simulink model "DSB_SSB"  (R2023a)
settings: Solver=VariableStepAuto  StartTime=0.0  StopTime=1  RelTol=1e-3
libraries: dspfdesign x2
settings Model: Creator=dung  LastModifiedBy=dung

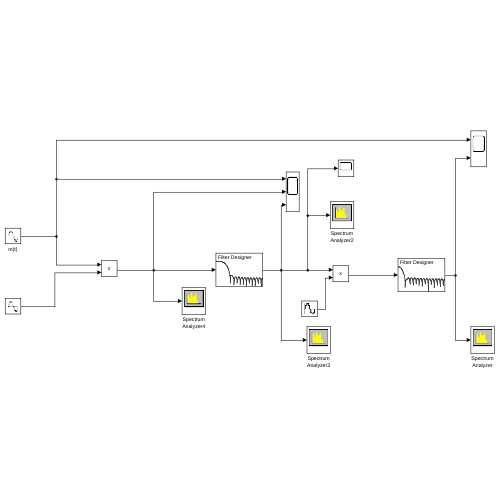
[thumbnail: Simulink's stored preview of the top-level diagram]
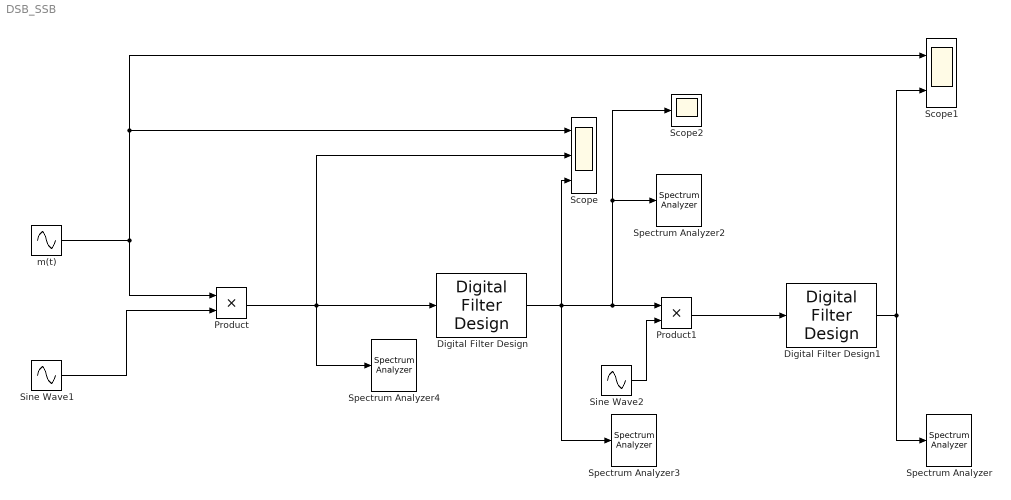
== system DSB_SSB ==
  Digital Filter Design : dspfdesign/Digital Filter Design  mwdsp_browser_bugfix_var=off
  Digital Filter Design1 : dspfdesign/Digital Filter Design  mwdsp_browser_bugfix_var=off
  Product : Product
  Product1 : Product
  Scope : Scope  NumInputPorts=3
  Scope1 : Scope  NumInputPorts=2
  Scope2 : Scope
  Sine Wave1 : Sin  Amplitude=5  Frequency=2*pi*10000  SampleTime=1/100000
  Sine Wave2 : Sin  Frequency=2*pi*10000  SampleTime=1/100000
  Spectrum Analyzer : SpectrumAnalyzer  WindowPosition=[560.000000,290.000000,800.000000,500.000000,]  ScopeFrameLocation=window  YLimits=[-253.6996542,53.22863961]  ColorLimits=[-20 80]  DefaultConfigurationName=spbscopes.SpectrumAnalyzerBlockCfg  IsFrequencyInputMode=0  FrequencyVectorPort=0  FrequencyVectorFromPort=0  FrequencyInputRBWPort=0  FrequencyInputRBWFromPort=0
  Spectrum Analyzer2 : SpectrumAnalyzer  WindowPosition=[562.000000,289.000000,800.000000,500.000000,]  ScopeFrameLocation=window  YLimits=[-248.57224363,56.6885393]  ColorLimits=[-20 80]  DefaultConfigurationName=spbscopes.SpectrumAnalyzerBlockCfg  IsFrequencyInputMode=0  FrequencyVectorPort=0  FrequencyVectorFromPort=0  FrequencyInputRBWPort=0  FrequencyInputRBWFromPort=0
  Spectrum Analyzer3 : SpectrumAnalyzer  WindowPosition=[1.000000,265.000000,1397.000000,752.000000,]  ScopeFrameLocation=window  YLimits=[-248.57224363,56.6885393]  ColorLimits=[-20 80]  DefaultConfigurationName=spbscopes.SpectrumAnalyzerBlockCfg  IsFrequencyInputMode=0  FrequencyVectorPort=0  FrequencyVectorFromPort=0  FrequencyInputRBWPort=0  FrequencyInputRBWFromPort=0
  Spectrum Analyzer4 : SpectrumAnalyzer  WindowPosition=[560.000000,290.000000,800.000000,500.000000,]  ScopeFrameLocation=window  Span=99999.99999999999  StartFrequency=-49999.99999999999  StopFrequency=49999.99999999999  YLimits=[-196.25019051,57.2918176]  ColorLimits=[-20 80]  DefaultConfigurationName=spbscopes.SpectrumAnalyzerBlockCfg  IsFrequencyInputMode=0  FrequencyVectorPort=0  FrequencyVectorFromPort=0  FrequencyInputRBWPort=0  FrequencyInputRBWFromPort=0
  m(t) : Sin  Frequency=2*pi*1000  SampleTime=1/100000
  wires:
  m(t)/1 -> Product/1, Scope1/1, Scope/1
  Digital Filter Design/1 -> Scope2/1, Spectrum Analyzer2/1, Product1/1, Spectrum Analyzer3/1, Scope/3
  Digital Filter Design1/1 -> Spectrum Analyzer/1, Scope1/2
  Sine Wave1/1 -> Product/2
  Product1/1 -> Digital Filter Design1/1
  Sine Wave2/1 -> Product1/2
  Product/1 -> Spectrum Analyzer4/1, Scope/2, Digital Filter Design/1
